simulink model "DSPB_MMSE"  (Simulink 8.1)
settings: Solver=VariableStepDiscrete  StartTime=0.0  StopTime=DSPB_MMSE_param.endTime  RelTol=1e-3
PreLoadFcn:
  | % Run the setup script when the model is opened
  | setup_DSPB_MMSE;
InitFcn:
  | % Run the setup script again just before the
  | % model is run, so that any updates made
  | % after opening are applied.
  | setup_DSPB_MMSE;
  | %% DSPBuilder Start
  | alt_dspbuilder_update_model(bdroot)
  | %% DSPBuilder End
StartFcn:
  | %% DSPBuilder Start
  | alt_dspbuilder_hdlimport_prepare_for_simulation(bdroot)
  | %% DSPBuilder End
undefined symbols (not defined in the file or in its folder): a, AdvDSPBDMemDisplay, dpoly, DSPB_MMSE_param, dspba, evalAionMaskParam, pow, primtype, UseDontCare, value, x, y
libraries: DSPBAPrim x213, DspbAdvFftLibrary x9, DSPBABase x5, simulink x3, DSPBAModelBus x3, DSPBAControl x1, DSPBAVectorUtil x1
(part 2 of 3)

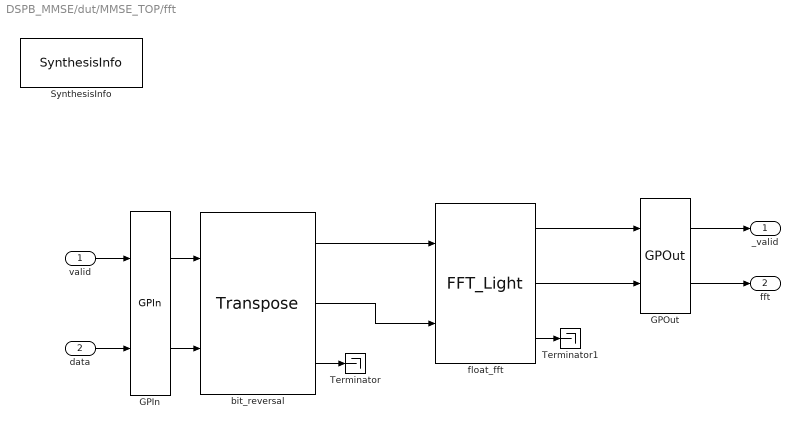
== system DSPB_MMSE/dut/MMSE_TOP/fft ==
  valid : Inport
  data : Inport  Port=2
  GPIn : DSPBAPrim/GPIn  primtype=gpin  nInputs=evalAionMaskParam(gcb,'value',1)  nOutputs=evalAionMaskParam(gcb,'value',1)  omode=Inherit via internal rule  otype=sfix(16)  scale=2^-15  rndmethod=Unbiased  factor=1  satmethod=Symmetric  shift_vec=[0 1 2 -1]  value=2  inPortNames=[' ' ' ' ' ' ' ' ' ' ' ' ' ' ' ' ' ' ' ' ' ' ' ' ' ' ' ' ' ' ' ' ' ' ' ' ' ' ' ' ' ' ' ' ' ' ' ' ' ' ' ' ' ' ' ' ' ' ' ' ' ' ' ' ' ' ' ' ' ']'  outPortNames=[' ' ' ' ' ' ' ' ' ' ' ' ' ' ' ' ' ' ' ' ' ' ' ' ' ' ' ' ' ' ' ' ' ' ' ' ' ' ' ' ' ' ' ' ' ' ' ' ' ' ' ' ' ' ' ' ' ' ' ' ' ' ' ' ' ' ' ' ' ']'  dspbaimage=dspba_prim.jpg  text=fprintf('GPIn');  style=Optimised  visibilities=1024  latencyCorrection=0  scheduleOrigin=on  version=20090407
  GPOut : DSPBAPrim/GPOut  primtype=gpout  nInputs=evalAionMaskParam(gcb,'value',1)  nOutputs=evalAionMaskParam(gcb,'value',1)  omode=Inherit via internal rule  otype=sfix(16)  scale=2^-15  rndmethod=Unbiased  factor=1  satmethod=Symmetric  shift_vec=[0 1 2 -1]  value=2  inPortNames=[' ' ' ' ' ' ' ' ' ' ' ' ' ' ' ' ' ' ' ' ' ' ' ' ' ' ' ' ' ' ' ' ' ' ' ' ' ' ' ' ' ' ' ' ' ' ' ' ' ' ' ' ' ' ' ' ' ' ' ' ' ' ' ' ' ' ' ' ' ']'  outPortNames=[' ' ' ' ' ' ' ' ' ' ' ' ' ' ' ' ' ' ' ' ' ' ' ' ' ' ' ' ' ' ' ' ' ' ' ' ' ' ' ' ' ' ' ' ' ' ' ' ' ' ' ' ' ' ' ' ' ' ' ' ' ' ' ' ' ' ' ' ' ']'  dspbaimage=dspba_prim.jpg  text=fprintf('GPOut');  style=Optimised  visibilities=1024  latencyCorrection=0  version=20090407
  SynthesisInfo : DSPBAPrim/SynthesisInfo  primtype=synthinfo  nInputs=0  nOutputs=0  omode=Inherit via internal rule  otype=sfix(16)  scale=2^-15  rndmethod=Truncate  factor=1  satmethod=Symmetric  shift_vec=[0 1 2 -1]  value=99  inPortNames=[' '; ' ';]  outPortNames=[' ']  dspbaimage=dspba_prim_ctrl.jpg  text=fprintf('Style=%s', style);  style=Scheduled  visibilities=32768  constraintInUse=off  constraintRelation=>  constraintLimit=2  bitAccurate=on  version=20150220
  Terminator : Terminator
  Terminator1 : Terminator
  bit_reversal : DspbAdvFftLibrary/Common/Transpose  perm=[fliplr(0:DSPB_MMSE_param.FS-1)]
  float_fft : DspbAdvFftLibrary/Common/FFT_Light  IFFT=false  subchannels=1  br_in=true  N=DSPB_MMSE_param.FS  in_type=dspba.namedVPFloat('single')  type_strings=dspba.fft.all_float(DSPB_MMSE_param.FS,dspba.namedVPFloat('single'))  faithful=false  wirecount=1
  _valid : Outport
  fft : Outport  Port=2
  wires:
  bit_reversal/3 -> Terminator/1
  bit_reversal/1 -> float_fft/1
  bit_reversal/2 -> float_fft/2
  float_fft/3 -> Terminator1/1
  GPIn/1 -> bit_reversal/1
  GPIn/2 -> bit_reversal/2
  valid/1 -> GPIn/1
  data/1 -> GPIn/2
  GPOut/1 -> _valid/1
  GPOut/2 -> fft/1
  float_fft/1 -> GPOut/1
  float_fft/2 -> GPOut/2

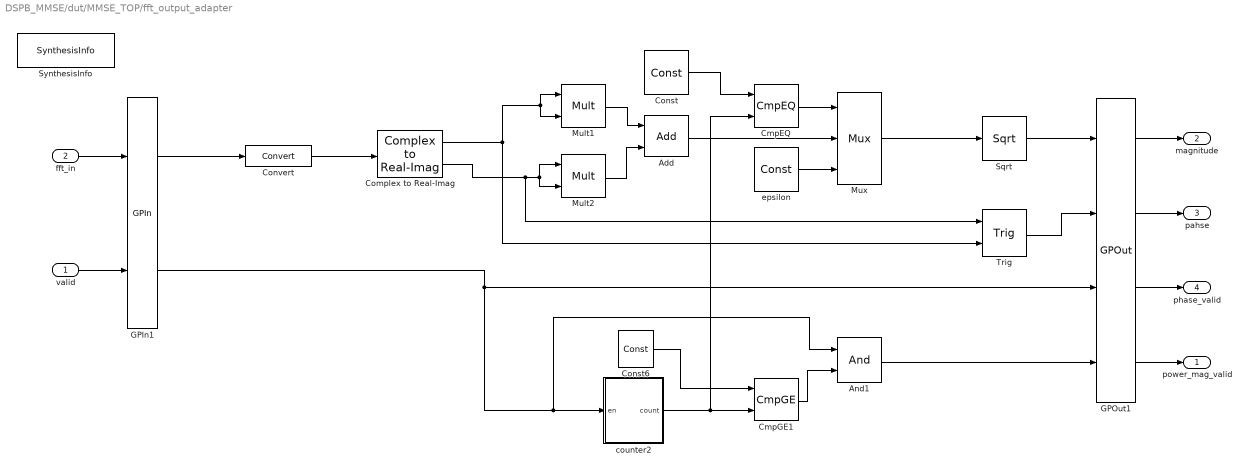
== system DSPB_MMSE/dut/MMSE_TOP/fft_output_adapter ==
  valid : Inport
  fft_in : Inport  Port=2
  Add : DSPBAPrim/Add  primtype=add  nInputs=evalAionMaskParam(gcb,'value',1)  nOutputs=1  omode=Inherit via internal rule with word growth  otype=sfix(16)  scale=2^-15  rndmethod=Unbiased  factor=1  satmethod=Symmetric  shift_vec=[0 1 2 -1]  value=2  inPortNames=[' '; ' ';]  outPortNames=[' ']  dspbaimage=dspba_prim.jpg  text=fprintf('+');  style=Optimised  visibilities=1032+2^17+2^18+2^19  genFPC=off  floatRounding=correct  advOptions=[]  version=20130821
  And1 : DSPBAPrim/And  primtype=and  nInputs=2  nOutputs=1  omode=Inherit via internal rule  otype=sfix(16)  scale=2^-15  rndmethod=Unbiased  factor=1  satmethod=Symmetric  shift_vec=[0 1 2 -1]  value=0  inPortNames=[' '; ' '; ' '; ' '; ' '; ' '; ' '; ' '; ' '; ' '; ' '; ' '; ' '; ' '; ' '; ' '; ]  outPortNames=[' ']  dspbaimage=dspba_prim.jpg  text=fprintf('&');  style=Optimised  visibilities=8+2  version=20090407
  CmpEQ : DSPBAPrim/CmpEQ  primtype=cmpeq  nInputs=2  nOutputs=1  omode=boolean  otype=sfix(16)  scale=2^-15  rndmethod=Unbiased  factor=1  satmethod=Symmetric  shift_vec=[0 1 2 -1]  value=0  inPortNames=[' '; ' ';]  outPortNames=[' ']  dspbaimage=dspba_prim.jpg  text=fprintf('==');  style=Optimised  visibilities=0  advOptions=[]  version=20130117
  CmpGE1 : DSPBAPrim/CmpGE  primtype=cmpgte  nInputs=2  nOutputs=1  omode=boolean  otype=sfix(16)  scale=2^-15  rndmethod=Unbiased  factor=1  satmethod=Symmetric  shift_vec=[0 1 2 -1]  value=0  inPortNames=['a'; 'b';]  outPortNames=[' ']  dspbaimage=dspba_prim.jpg  text=fprintf('a>=b');  style=Optimised  visibilities=0  advOptions=[]  version=20130117
  Complex to Real-Imag : DSPBAVectorUtil/Complex to Real-Imag
  Const : DSPBAPrim/Const  primtype=const  nInputs=0  nOutputs=1  omode=Inherit via internal rule  otype=sfix(16)  scale=2^-15  rndmethod=Unbiased  factor=1  satmethod=Symmetric  shift_vec=[0 1 2 -1]  value=1  inPortNames=['+'; '+';]  outPortNames=[' ']  dspbaimage=dspba_prim.jpg  text=fprintf('%s', num2str(value));  style=Optimised  visibilities=8 + 1024  floatPrecision=float32_m23  version=20120820
  Const6 : DSPBAPrim/Const  primtype=const  nInputs=0  nOutputs=1  omode=Specify via dialog  otype=ufix(DSPB_MMSE_param.FS+1)  scale=2^-0  rndmethod=Unbiased  factor=1  satmethod=Symmetric  shift_vec=[0 1 2 -1]  value=2^(DSPB_MMSE_param.FS-1)  inPortNames=['+'; '+';]  outPortNames=[' ']  dspbaimage=dspba_prim.jpg  text=fprintf('%s', num2str(value));  style=Optimised  visibilities=8 + 1024  floatPrecision=float32_m23  version=20120820
  Convert : DSPBAPrim/Convert  primtype=convert  nInputs=1  nOutputs=1  omode=single  otype=sfix(16)  scale=2^-15  rndmethod=Biased  factor=1  satmethod=None  shift_vec=[0 1 2 -1]  value=round([0:255]/17)  inPortNames=[' '; ' ';]  outPortNames=[' '; 'c']  dspbaimage=dspba_prim.jpg  text=fprintf('convert');  style=Optimised  visibilities=8+64+256+2^17  clipdetect=off  floatPrecision=float32_m23  advOptions=[]  version=20130211
  GPIn1 : DSPBAPrim/GPIn  primtype=gpin  nInputs=evalAionMaskParam(gcb,'value',1)  nOutputs=evalAionMaskParam(gcb,'value',1)  omode=Inherit via internal rule  otype=sfix(16)  scale=2^-15  rndmethod=Unbiased  factor=1  satmethod=Symmetric  shift_vec=[0 1 2 -1]  value=2  inPortNames=[' ' ' ' ' ' ' ' ' ' ' ' ' ' ' ' ' ' ' ' ' ' ' ' ' ' ' ' ' ' ' ' ' ' ' ' ' ' ' ' ' ' ' ' ' ' ' ' ' ' ' ' ' ' ' ' ' ' ' ' ' ' ' ' ' ' ' ' ' ']'  outPortNames=[' ' ' ' ' ' ' ' ' ' ' ' ' ' ' ' ' ' ' ' ' ' ' ' ' ' ' ' ' ' ' ' ' ' ' ' ' ' ' ' ' ' ' ' ' ' ' ' ' ' ' ' ' ' ' ' ' ' ' ' ' ' ' ' ' ' ' ' ' ']'  dspbaimage=dspba_prim.jpg  text=fprintf('GPIn');  style=Optimised  visibilities=1024  latencyCorrection=0  scheduleOrigin=on  version=20090407
  GPOut1 : DSPBAPrim/GPOut  primtype=gpout  nInputs=evalAionMaskParam(gcb,'value',1)  nOutputs=evalAionMaskParam(gcb,'value',1)  omode=Inherit via internal rule  otype=sfix(16)  scale=2^-15  rndmethod=Unbiased  factor=1  satmethod=Symmetric  shift_vec=[0 1 2 -1]  value=4  inPortNames=[' ' ' ' ' ' ' ' ' ' ' ' ' ' ' ' ' ' ' ' ' ' ' ' ' ' ' ' ' ' ' ' ' ' ' ' ' ' ' ' ' ' ' ' ' ' ' ' ' ' ' ' ' ' ' ' ' ' ' ' ' ' ' ' ' ' ' ' ' ']'  outPortNames=[' ' ' ' ' ' ' ' ' ' ' ' ' ' ' ' ' ' ' ' ' ' ' ' ' ' ' ' ' ' ' ' ' ' ' ' ' ' ' ' ' ' ' ' ' ' ' ' ' ' ' ' ' ' ' ' ' ' ' ' ' ' ' ' ' ' ' ' ' ']'  dspbaimage=dspba_prim.jpg  text=fprintf('GPOut');  style=Optimised  visibilities=1024  latencyCorrection=0  version=20090407
  Mult1 : DSPBAPrim/Mult  primtype=mult  nInputs=2  nOutputs=1  omode=Inherit via internal rule  otype=sfix(16)  scale=2^-15  rndmethod=Unbiased  factor=1  satmethod=Symmetric  shift_vec=[0 1 2 -1]  value=0  inPortNames=[' '; ' ';]  outPortNames=[' ']  dspbaimage=dspba_prim.jpg  text=fprintf('X');  style=Optimised  visibilities=8+2^18+2^19  floatPrecision=float32_m23  floatRounding=correct  advOptions=[]  version=20130115
  Mult2 : DSPBAPrim/Mult  primtype=mult  nInputs=2  nOutputs=1  omode=Inherit via internal rule  otype=sfix(16)  scale=2^-15  rndmethod=Unbiased  factor=1  satmethod=Symmetric  shift_vec=[0 1 2 -1]  value=0  inPortNames=[' '; ' ';]  outPortNames=[' ']  dspbaimage=dspba_prim.jpg  text=fprintf('X');  style=Optimised  visibilities=8+2^18+2^19  floatPrecision=float32_m23  floatRounding=correct  advOptions=[]  version=20130115
  Mux : DSPBAPrim/Mux  primtype=mux  nInputs=evalAionMaskParam(gcb,'value',1)+1  nOutputs=1  omode=Inherit via internal rule  otype=sfix(16)  scale=2^-15  rndmethod=Unbiased  factor=1  satmethod=Symmetric  shift_vec=[0 1 2 -1]  value=2  inPortNames=['s '; 'd0'; 'd1'; 'd2'; 'd3'; 'd4'; 'd5'; 'd6'; 'd7'; 'd8'; 'd9';]  outPortNames=[' ']  dspbaimage=dspba_prim.jpg  text=fprintf('%s', primtype);  style=Optimised  visibilities=1032  version=20131025
  Sqrt : DSPBAPrim/Sqrt  primtype=sqrtfunc  nInputs=1  nOutputs=1  omode=Inherit via internal rule  otype=sfix(16)  scale=2^-15  rndmethod=Unbiased  factor=1  satmethod=Symmetric  shift_vec=[0 1 2 -1]  value=round([0:255]/17)  inPortNames=[' '; ' ';]  outPortNames=[' ']  dspbaimage=dspba_prim_float.jpg  text=fprintf('sqrt(x)');  style=Optimised  visibilities=2^17  functionExpr=sqrt(x)  floatRounding=correct  advOptions=[]  version=20120730
  SynthesisInfo : DSPBAPrim/SynthesisInfo  primtype=synthinfo  nInputs=0  nOutputs=0  omode=Inherit via internal rule  otype=sfix(16)  scale=2^-15  rndmethod=Truncate  factor=1  satmethod=Symmetric  shift_vec=[0 1 2 -1]  value=99  inPortNames=[' '; ' ';]  outPortNames=[' ']  dspbaimage=dspba_prim_ctrl.jpg  text=fprintf('Style=%s', style);  style=Scheduled  visibilities=2^17+2^18+2^19+2^20  constraintInUse=off  constraintRelation=>  constraintLimit=2  bitAccurate=on  version=20150220
  Trig : DSPBAPrim/Trig  primtype=trigfunc  nInputs=1  nOutputs=1  omode=Inherit via internal rule  otype=sfix(16)  scale=2^-15  rndmethod=Unbiased  factor=1  satmethod=Symmetric  shift_vec=[0 1 2 -1]  value=round([0:255]/17)  inPortNames=[' '; ' ';]  outPortNames=[' ']  dspbaimage=dspba_prim_float.jpg  text=fprintf('sin(a)');  style=Optimised  visibilities=2^17+2^18  functionExpr=atan2(y;x)  advOptions=[]  version=20140803
  counter2 : Subsystem
  epsilon : DSPBAPrim/Const  primtype=const  nInputs=0  nOutputs=1  omode=single  otype=sfix(16)  scale=2^-15  rndmethod=Unbiased  factor=1  satmethod=Symmetric  shift_vec=[0 1 2 -1]  value=2^-126  inPortNames=['+'; '+';]  outPortNames=[' ']  dspbaimage=dspba_prim.jpg  text=fprintf('%s', num2str(value));  style=Optimised  visibilities=8 + 1024  floatPrecision=float32_m23  version=20120820
  power_mag_valid : Outport
  magnitude : Outport  Port=2
  pahse : Outport  Port=3
  phase_valid : Outport  Port=4
  wires:
  Mult1/1 -> Add/1
  Mult2/1 -> Add/2
  GPOut1/1 -> magnitude/1
  valid/1 -> GPIn1/2
  fft_in/1 -> GPIn1/1
  GPIn1/1 -> Convert/1
  GPOut1/2 -> pahse/1
  Complex to Real-Imag/1 -> Mult1/2, Mult1/1, Trig/2
  Complex to Real-Imag/2 -> Trig/1, Mult2/2, Mult2/1
  GPOut1/3 -> phase_valid/1
  Trig/1 -> GPOut1/2
  GPIn1/2 -> counter2/1(en), And1/1, GPOut1/3
  Const6/1 -> CmpGE1/1
  counter2/1(count) -> CmpEQ/2, CmpGE1/2
  CmpGE1/1 -> And1/2
  And1/1 -> GPOut1/4
  GPOut1/4 -> power_mag_valid/1
  Mux/1 -> Sqrt/1
  Sqrt/1 -> GPOut1/1
  Convert/1 -> Complex to Real-Imag/1
  Const/1 -> CmpEQ/1
  CmpEQ/1 -> Mux/1
  Add/1 -> Mux/2
  epsilon/1 -> Mux/3

== system DSPB_MMSE/dut/MMSE_TOP/reconstruct ==
  valid : Inport
  enhanced_mag : Inport  Port=2
  phase : Inport  Port=3
  pahse_valid : Inport  Port=4
  ifft : Subsystem
  ifft_input_adapter : Subsystem
  _valid : Outport
  output : Outport  Port=2
  wires:
  ifft/2(ifft) -> output/1
  valid/1 -> ifft_input_adapter/2(valid)
  ifft/1(_valid) -> _valid/1
  ifft_input_adapter/1(_valid) -> ifft/1(valid)
  ifft_input_adapter/2(out) -> ifft/2(data)
  enhanced_mag/1 -> ifft_input_adapter/3(enhanced_mag)
  pahse_valid/1 -> ifft_input_adapter/1(phase_valid)
  phase/1 -> ifft_input_adapter/4(phase)

== system DSPB_MMSE/dut/MM_in/addr_counter ==
  en : Inport
  CmpEQ : DSPBAPrim/CmpEQ  primtype=cmpeq  nInputs=2  nOutputs=1  omode=boolean  otype=sfix(16)  scale=2^-15  rndmethod=Unbiased  factor=1  satmethod=Symmetric  shift_vec=[0 1 2 -1]  value=0  inPortNames=[' '; ' ';]  outPortNames=[' ']  dspbaimage=dspba_prim.jpg  text=fprintf('==');  style=Optimised  visibilities=0  advOptions=[]  version=20130117
  Const1 : DSPBAPrim/Const  primtype=const  nInputs=0  nOutputs=1  omode=Specify via dialog  otype=ufix(DSPB_MMSE_param.FS+1)  scale=2^-0  rndmethod=Unbiased  factor=1  satmethod=Symmetric  shift_vec=[0 1 2 -1]  value=2^(DSPB_MMSE_param.FS) + 1  inPortNames=['+'; '+';]  outPortNames=[' ']  dspbaimage=dspba_prim.jpg  text=fprintf('%s', num2str(value));  style=Optimised  visibilities=8 + 1024  floatPrecision=float32_m23  version=20120820
  Const2 : DSPBAPrim/Const  primtype=const  nInputs=0  nOutputs=1  omode=Specify via dialog  otype=ufix(DSPB_MMSE_param.FS + 1)  scale=2^-0  rndmethod=Unbiased  factor=1  satmethod=Symmetric  shift_vec=[0 1 2 -1]  value=2^(DSPB_MMSE_param.FS)  inPortNames=['+'; '+';]  outPortNames=[' ']  dspbaimage=dspba_prim.jpg  text=fprintf('%s', num2str(value));  style=Optimised  visibilities=8 + 1024  floatPrecision=float32_m23  version=20120820
  Const3 : DSPBAPrim/Const  primtype=const  nInputs=0  nOutputs=1  omode=boolean  otype=ufix(10)  scale=2^-0  rndmethod=Unbiased  factor=1  satmethod=Symmetric  shift_vec=[0 1 2 -1]  value=1  inPortNames=['+'; '+';]  outPortNames=[' ']  dspbaimage=dspba_prim.jpg  text=fprintf('%s', num2str(value));  style=Optimised  visibilities=8 + 1024  floatPrecision=float32_m23  version=20120820
  Const4 : DSPBAPrim/Const  primtype=const  nInputs=0  nOutputs=1  omode=Inherit via internal rule  otype=ufix(10)  scale=2^-0  rndmethod=Unbiased  factor=1  satmethod=Symmetric  shift_vec=[0 1 2 -1]  value=0  inPortNames=['+'; '+';]  outPortNames=[' ']  dspbaimage=dspba_prim.jpg  text=fprintf('%s', num2str(value));  style=Optimised  visibilities=8 + 1024  floatPrecision=float32_m23  version=20120820
  LoadableCounter : DSPBAPrim/LoadableCounter  primtype=loadablecounter  nInputs=5  nOutputs=1  omode=Specify via dialog  otype=ufix(DSPB_MMSE_param.FS+1)  scale=2^-0  rndmethod=Unbiased  factor=1  satmethod=Symmetric  shift_vec=[0 1 2 -1]  value=[0 2^(DSPB_MMSE_param.FS) + 1 1]  inPortNames=['en';'ld';'i ';'s ';'m ']  outPortNames=[' ']  dspbaimage=dspba_prim.jpg  text=fprintf('loadable\ncounter\n[%d %d %d]', value(1), value(2), value(3));  style=Optimised  visibilities=8 + 1024  version=20090407
  SampleDelay : DSPBAPrim/SampleDelay  primtype=sampdelay  nInputs=1  nOutputs=1  omode=Inherit via internal rule  otype=sfix(16)  scale=2^-15  rndmethod=Unbiased  factor=1  satmethod=Symmetric  shift_vec=[0 1 2 -1]  value=1  inPortNames=[' '; ' ';]  outPortNames=[' ']  dspbaimage=dspba_prim.jpg  text=dpoly(1, eye(1,value+1), 'z')  style=Optimised  visibilities=8 + 1024 + 2^17 + 2^18  flexible=off  slackgroup=0  augmented=0  version=20090407  advOptions=[]
  count : Outport
  wires:
  Const2/1 -> CmpEQ/2
  CmpEQ/1 -> SampleDelay/1
  Const4/1 -> LoadableCounter/3
  Const1/1 -> LoadableCounter/5
  SampleDelay/1 -> LoadableCounter/2
  Const3/1 -> LoadableCounter/4
  en/1 -> LoadableCounter/1
  LoadableCounter/1 -> count/1, CmpEQ/1

== system DSPB_MMSE/dut/MM_out/addr_counter1 ==
  en : Inport
  CmpEQ : DSPBAPrim/CmpEQ  primtype=cmpeq  nInputs=2  nOutputs=1  omode=boolean  otype=sfix(16)  scale=2^-15  rndmethod=Unbiased  factor=1  satmethod=Symmetric  shift_vec=[0 1 2 -1]  value=0  inPortNames=[' '; ' ';]  outPortNames=[' ']  dspbaimage=dspba_prim.jpg  text=fprintf('==');  style=Optimised  visibilities=0  advOptions=[]  version=20130117
  Const1 : DSPBAPrim/Const  primtype=const  nInputs=0  nOutputs=1  omode=Specify via dialog  otype=ufix(DSPB_MMSE_param.FS+1)  scale=2^-0  rndmethod=Unbiased  factor=1  satmethod=Symmetric  shift_vec=[0 1 2 -1]  value=2^(DSPB_MMSE_param.FS) + 1  inPortNames=['+'; '+';]  outPortNames=[' ']  dspbaimage=dspba_prim.jpg  text=fprintf('%s', num2str(value));  style=Optimised  visibilities=8 + 1024  floatPrecision=float32_m23  version=20120820
  Const2 : DSPBAPrim/Const  primtype=const  nInputs=0  nOutputs=1  omode=Specify via dialog  otype=ufix(DSPB_MMSE_param.FS + 1)  scale=2^-0  rndmethod=Unbiased  factor=1  satmethod=Symmetric  shift_vec=[0 1 2 -1]  value=2^(DSPB_MMSE_param.FS)  inPortNames=['+'; '+';]  outPortNames=[' ']  dspbaimage=dspba_prim.jpg  text=fprintf('%s', num2str(value));  style=Optimised  visibilities=8 + 1024  floatPrecision=float32_m23  version=20120820
  Const3 : DSPBAPrim/Const  primtype=const  nInputs=0  nOutputs=1  omode=boolean  otype=ufix(10)  scale=2^-0  rndmethod=Unbiased  factor=1  satmethod=Symmetric  shift_vec=[0 1 2 -1]  value=1  inPortNames=['+'; '+';]  outPortNames=[' ']  dspbaimage=dspba_prim.jpg  text=fprintf('%s', num2str(value));  style=Optimised  visibilities=8 + 1024  floatPrecision=float32_m23  version=20120820
  Const4 : DSPBAPrim/Const  primtype=const  nInputs=0  nOutputs=1  omode=Inherit via internal rule  otype=ufix(10)  scale=2^-0  rndmethod=Unbiased  factor=1  satmethod=Symmetric  shift_vec=[0 1 2 -1]  value=0  inPortNames=['+'; '+';]  outPortNames=[' ']  dspbaimage=dspba_prim.jpg  text=fprintf('%s', num2str(value));  style=Optimised  visibilities=8 + 1024  floatPrecision=float32_m23  version=20120820
  LoadableCounter : DSPBAPrim/LoadableCounter  primtype=loadablecounter  nInputs=5  nOutputs=1  omode=Specify via dialog  otype=ufix(DSPB_MMSE_param.FS+1)  scale=2^-0  rndmethod=Unbiased  factor=1  satmethod=Symmetric  shift_vec=[0 1 2 -1]  value=[0 2^(DSPB_MMSE_param.FS) + 1 1]  inPortNames=['en';'ld';'i ';'s ';'m ']  outPortNames=[' ']  dspbaimage=dspba_prim.jpg  text=fprintf('loadable\ncounter\n[%d %d %d]', value(1), value(2), value(3));  style=Optimised  visibilities=8 + 1024  version=20090407
  SampleDelay : DSPBAPrim/SampleDelay  primtype=sampdelay  nInputs=1  nOutputs=1  omode=Inherit via internal rule  otype=sfix(16)  scale=2^-15  rndmethod=Unbiased  factor=1  satmethod=Symmetric  shift_vec=[0 1 2 -1]  value=1  inPortNames=[' '; ' ';]  outPortNames=[' ']  dspbaimage=dspba_prim.jpg  text=dpoly(1, eye(1,value+1), 'z')  style=Optimised  visibilities=8 + 1024 + 2^17 + 2^18  flexible=off  slackgroup=0  augmented=0  version=20090407  advOptions=[]
  count : Outport
  wires:
  Const2/1 -> CmpEQ/2
  CmpEQ/1 -> SampleDelay/1
  Const4/1 -> LoadableCounter/3
  Const1/1 -> LoadableCounter/5
  SampleDelay/1 -> LoadableCounter/2
  Const3/1 -> LoadableCounter/4
  en/1 -> LoadableCounter/1
  LoadableCounter/1 -> count/1, CmpEQ/1

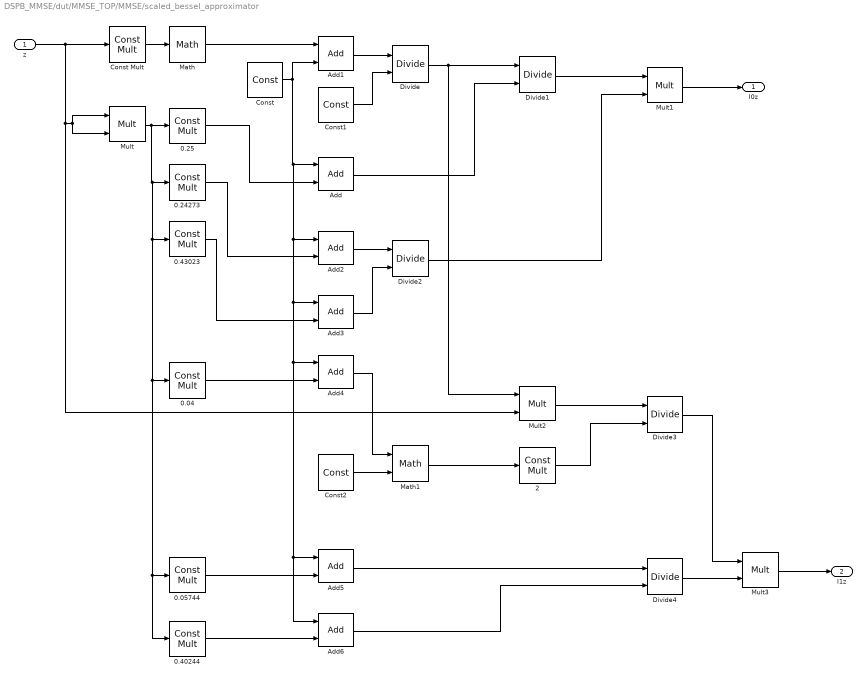
== system DSPB_MMSE/dut/MMSE_TOP/MMSE/scaled_bessel_approximator ==
  z : Inport
  0.04 : DSPBAPrim/Const Mult  primtype=constmult  nInputs=1  nOutputs=1  omode=Inherit via internal rule  otype=sfix(16)  scale=2^-15  rndmethod=Unbiased  factor=1  satmethod=Symmetric  shift_vec=[0 1 2 -1]  value=0.04  inPortNames=[' '; ' ';]  outPortNames=[' ']  dspbaimage=dspba_prim.jpg  text=fprintf('cx');  style=Optimised  visibilities=8+2^10+2^17+2^18  floatRounding=faithful  advOptions=[]  version=20140218
  0.05744 : DSPBAPrim/Const Mult  primtype=constmult  nInputs=1  nOutputs=1  omode=Inherit via internal rule  otype=sfix(16)  scale=2^-15  rndmethod=Unbiased  factor=1  satmethod=Symmetric  shift_vec=[0 1 2 -1]  value=0.05744  inPortNames=[' '; ' ';]  outPortNames=[' ']  dspbaimage=dspba_prim.jpg  text=fprintf('cx');  style=Optimised  visibilities=8+2^10+2^17+2^18  floatRounding=faithful  advOptions=[]  version=20140218
  0.24273 : DSPBAPrim/Const Mult  primtype=constmult  nInputs=1  nOutputs=1  omode=Inherit via internal rule  otype=sfix(16)  scale=2^-15  rndmethod=Unbiased  factor=1  satmethod=Symmetric  shift_vec=[0 1 2 -1]  value=0.24273  inPortNames=[' '; ' ';]  outPortNames=[' ']  dspbaimage=dspba_prim.jpg  text=fprintf('cx');  style=Optimised  visibilities=8+2^10+2^17+2^18  floatRounding=faithful  advOptions=[]  version=20140218
  0.25 : DSPBAPrim/Const Mult  primtype=constmult  nInputs=1  nOutputs=1  omode=Inherit via internal rule  otype=sfix(16)  scale=2^-15  rndmethod=Unbiased  factor=1  satmethod=Symmetric  shift_vec=[0 1 2 -1]  value=0.25  inPortNames=[' '; ' ';]  outPortNames=[' ']  dspbaimage=dspba_prim.jpg  text=fprintf('cx');  style=Optimised  visibilities=8+2^10+2^17+2^18  floatRounding=faithful  advOptions=[]  version=20140218
  0.40244 : DSPBAPrim/Const Mult  primtype=constmult  nInputs=1  nOutputs=1  omode=Inherit via internal rule  otype=sfix(16)  scale=2^-15  rndmethod=Unbiased  factor=1  satmethod=Symmetric  shift_vec=[0 1 2 -1]  value=0.40244  inPortNames=[' '; ' ';]  outPortNames=[' ']  dspbaimage=dspba_prim.jpg  text=fprintf('cx');  style=Optimised  visibilities=8+2^10+2^17+2^18  floatRounding=faithful  advOptions=[]  version=20140218
  0.43023 : DSPBAPrim/Const Mult  primtype=constmult  nInputs=1  nOutputs=1  omode=Inherit via internal rule  otype=sfix(16)  scale=2^-15  rndmethod=Unbiased  factor=1  satmethod=Symmetric  shift_vec=[0 1 2 -1]  value=0.43023  inPortNames=[' '; ' ';]  outPortNames=[' ']  dspbaimage=dspba_prim.jpg  text=fprintf('cx');  style=Optimised  visibilities=8+2^10+2^17+2^18  floatRounding=faithful  advOptions=[]  version=20140218
  2 : DSPBAPrim/Const Mult  primtype=constmult  nInputs=1  nOutputs=1  omode=Inherit via internal rule  otype=sfix(16)  scale=2^-15  rndmethod=Unbiased  factor=1  satmethod=Symmetric  shift_vec=[0 1 2 -1]  value=2  inPortNames=[' '; ' ';]  outPortNames=[' ']  dspbaimage=dspba_prim.jpg  text=fprintf('cx');  style=Optimised  visibilities=8+2^10+2^17+2^18  floatRounding=faithful  advOptions=[]  version=20140218
  Add{,1..6} (7 alike) : DSPBAPrim/Add  primtype=add  nInputs=evalAionMaskParam(gcb,'value',1)  nOutputs=1  omode=Inherit via internal rule with word growth  otype=sfix(16)  scale=2^-15  rndmethod=Unbiased  factor=1  satmethod=Symmetric  shift_vec=[0 1 2 -1]  value=2  inPortNames=[' '; ' ';]  outPortNames=[' ']  dspbaimage=dspba_prim.jpg  text=fprintf('+');  style=Optimised  visibilities=1032+2^17+2^18+2^19  genFPC=on  floatRounding=faithful  advOptions=[]  version=20130821
  Const : DSPBAPrim/Const  primtype=const  nInputs=0  nOutputs=1  omode=single  otype=sfix(16)  scale=2^-15  rndmethod=Unbiased  factor=1  satmethod=Symmetric  shift_vec=[0 1 2 -1]  value=1  inPortNames=['+'; '+';]  outPortNames=[' ']  dspbaimage=dspba_prim.jpg  text=fprintf('%s', num2str(value));  style=Optimised  visibilities=8 + 1024  floatPrecision=float32_m23  version=20120820
  Const Mult : DSPBAPrim/Const Mult  primtype=constmult  nInputs=1  nOutputs=1  omode=Inherit via internal rule  otype=sfix(16)  scale=2^-15  rndmethod=Unbiased  factor=1  satmethod=Symmetric  shift_vec=[0 1 2 -1]  value=-2  inPortNames=[' '; ' ';]  outPortNames=[' ']  dspbaimage=dspba_prim.jpg  text=fprintf('cx');  style=Optimised  visibilities=8+2^10+2^17+2^18  floatRounding=faithful  advOptions=[]  version=20140218
  Const1 : DSPBAPrim/Const  primtype=const  nInputs=0  nOutputs=1  omode=single  otype=sfix(16)  scale=2^-15  rndmethod=Unbiased  factor=1  satmethod=Symmetric  shift_vec=[0 1 2 -1]  value=2  inPortNames=['+'; '+';]  outPortNames=[' ']  dspbaimage=dspba_prim.jpg  text=fprintf('%s', num2str(value));  style=Optimised  visibilities=8 + 1024  floatPrecision=float32_m23  version=20120820
  Const2 : DSPBAPrim/Const  primtype=const  nInputs=0  nOutputs=1  omode=single  otype=sfix(16)  scale=2^-15  rndmethod=Unbiased  factor=1  satmethod=Symmetric  shift_vec=[0 1 2 -1]  value=3/4  inPortNames=['+'; '+';]  outPortNames=[' ']  dspbaimage=dspba_prim.jpg  text=fprintf('%s', num2str(value));  style=Optimised  visibilities=8 + 1024  floatPrecision=float32_m23  version=20120820
  Divide{,1..4} (5 alike) : DSPBAPrim/Divide  primtype=divide  nInputs=2  nOutputs=1  omode=Inherit via internal rule  otype=sfix(16)  scale=2^-15  rndmethod=Unbiased  factor=1  satmethod=Symmetric  shift_vec=[0 1 2 -1]  value=round([0:255]/17)  inPortNames=[' '; ' ';]  outPortNames=[' ']  dspbaimage=dspba_prim.jpg  text=fprintf('a\n----\nb');  style=Optimised  visibilities=8+2^17+2^18  floatRounding=faithful  advOptions=[]  version=20130115
  Math : DSPBAPrim/Math  primtype=mathfunc  nInputs=1  nOutputs=1  omode=Inherit via internal rule  otype=sfix(16)  scale=2^-15  rndmethod=Unbiased  factor=1  satmethod=Symmetric  shift_vec=[0 1 2 -1]  value=round([0:255]/17)  inPortNames=[' '; ' ';]  outPortNames=[' ']  dspbaimage=dspba_prim_float.jpg  text=fprintf('exp(x)');  style=Optimised  visibilities=2^17  functionExpr=exp(x)  advOptions=[]  floatRounding=correct  version=20130910
  Math1 : DSPBAPrim/Math  primtype=mathfunc  nInputs=1  nOutputs=1  omode=Inherit via internal rule  otype=sfix(16)  scale=2^-15  rndmethod=Unbiased  factor=1  satmethod=Symmetric  shift_vec=[0 1 2 -1]  value=round([0:255]/17)  inPortNames=[' '; ' ';]  outPortNames=[' ']  dspbaimage=dspba_prim_float.jpg  text=fprintf('exp(x)');  style=Optimised  visibilities=2^17  functionExpr=pow(x;y)  advOptions=[]  floatRounding=correct  version=20130910
  Mult{,1..3} (4 alike) : DSPBAPrim/Mult  primtype=mult  nInputs=2  nOutputs=1  omode=Inherit via internal rule  otype=sfix(16)  scale=2^-15  rndmethod=Unbiased  factor=1  satmethod=Symmetric  shift_vec=[0 1 2 -1]  value=0  inPortNames=[' '; ' ';]  outPortNames=[' ']  dspbaimage=dspba_prim.jpg  text=fprintf('X');  style=Optimised  visibilities=8+2^18+2^19  floatPrecision=float32_m23  floatRounding=faithful  advOptions=[]  version=20130115
  I0z : Outport
  I1z : Outport  Port=2
  wires:
  z/1 -> Mult2/2, Mult/2, Mult/1, Const Mult/1
  Const Mult/1 -> Math/1
  Const/1 -> Add1/2, Add6/1, Add5/1, Add4/1, Add3/1, Add2/1, Add/1
  Math/1 -> Add1/1
  Add1/1 -> Divide/1
  Const1/1 -> Divide/2
  Divide/1 -> Mult2/1, Divide1/1
  Mult/1 -> 0.40244/1, 0.05744/1, 0.04/1, 0.43023/1, 0.24273/1, 0.25/1
  0.25/1 -> Add/2
  Add/1 -> Divide1/2
  Divide1/1 -> Mult1/1
  0.24273/1 -> Add2/2
  Add2/1 -> Divide2/1
  0.43023/1 -> Add3/2
  Add3/1 -> Divide2/2
  Divide2/1 -> Mult1/2
  Mult1/1 -> I0z/1
  Mult2/1 -> Divide3/1
  0.04/1 -> Add4/2
  Add4/1 -> Math1/1
  Const2/1 -> Math1/2
  Math1/1 -> 2/1
  2/1 -> Divide3/2
  Divide3/1 -> Mult3/1
  Divide4/1 -> Mult3/2
  0.05744/1 -> Add5/2
  0.40244/1 -> Add6/2
  Add5/1 -> Divide4/1
  Add6/1 -> Divide4/2
  Mult3/1 -> I1z/1

== system DSPB_MMSE/dut/MMSE_TOP/MMSE/v_k ==
  a_priori_snr : Inport
  a_posteriori_snr : Inport  Port=2
  Add : DSPBAPrim/Add  primtype=add  nInputs=evalAionMaskParam(gcb,'value',1)  nOutputs=1  omode=Inherit via internal rule with word growth  otype=sfix(16)  scale=2^-15  rndmethod=Unbiased  factor=1  satmethod=Symmetric  shift_vec=[0 1 2 -1]  value=2  inPortNames=[' '; ' ';]  outPortNames=[' ']  dspbaimage=dspba_prim.jpg  text=fprintf('+');  style=Optimised  visibilities=1032+2^17+2^18+2^19  genFPC=off  floatRounding=correct  advOptions=[]  version=20130821
  Const1 : DSPBAPrim/Const  primtype=const  nInputs=0  nOutputs=1  omode=single  otype=sfix(16)  scale=2^-15  rndmethod=Unbiased  factor=1  satmethod=Symmetric  shift_vec=[0 1 2 -1]  value=1  inPortNames=['+'; '+';]  outPortNames=[' ']  dspbaimage=dspba_prim.jpg  text=fprintf('%s', num2str(value));  style=Optimised  visibilities=8 + 1024  floatPrecision=float32_m23  version=20120820
  Divide1 : DSPBAPrim/Divide  primtype=divide  nInputs=2  nOutputs=1  omode=Inherit via internal rule  otype=sfix(16)  scale=2^-15  rndmethod=Unbiased  factor=1  satmethod=Symmetric  shift_vec=[0 1 2 -1]  value=round([0:255]/17)  inPortNames=[' '; ' ';]  outPortNames=[' ']  dspbaimage=dspba_prim.jpg  text=fprintf('a\n----\nb');  style=Optimised  visibilities=8+2^17+2^18  floatRounding=correct  advOptions=[]  version=20130115
  Mult1 : DSPBAPrim/Mult  primtype=mult  nInputs=2  nOutputs=1  omode=Inherit via internal rule  otype=sfix(16)  scale=2^-15  rndmethod=Unbiased  factor=1  satmethod=Symmetric  shift_vec=[0 1 2 -1]  value=0  inPortNames=[' '; ' ';]  outPortNames=[' ']  dspbaimage=dspba_prim.jpg  text=fprintf('X');  style=Optimised  visibilities=8+2^18+2^19  floatPrecision=float32_m23  floatRounding=correct  advOptions=[]  version=20130115
  v_k : Outport
  wires:
  a_priori_snr/1 -> Divide1/1, Add/1
  Const1/1 -> Add/2
  a_posteriori_snr/1 -> Mult1/2
  Add/1 -> Divide1/2
  Divide1/1 -> Mult1/1
  Mult1/1 -> v_k/1

== system DSPB_MMSE/dut/MMSE_TOP/a_posteriori_snr/counter ==
  en : Inport
  CmpEQ : DSPBAPrim/CmpEQ  primtype=cmpeq  nInputs=2  nOutputs=1  omode=boolean  otype=sfix(16)  scale=2^-15  rndmethod=Unbiased  factor=1  satmethod=Symmetric  shift_vec=[0 1 2 -1]  value=0  inPortNames=[' '; ' ';]  outPortNames=[' ']  dspbaimage=dspba_prim.jpg  text=fprintf('==');  style=Optimised  visibilities=0  advOptions=[]  version=20130117
  Const1 : DSPBAPrim/Const  primtype=const  nInputs=0  nOutputs=1  omode=Specify via dialog  otype=ufix(DSPB_MMSE_param.FS+1)  scale=2^-0  rndmethod=Unbiased  factor=1  satmethod=Symmetric  shift_vec=[0 1 2 -1]  value=2^(DSPB_MMSE_param.FS-1)+1  inPortNames=['+'; '+';]  outPortNames=[' ']  dspbaimage=dspba_prim.jpg  text=fprintf('%s', num2str(value));  style=Optimised  visibilities=8 + 1024  floatPrecision=float32_m23  version=20120820
  Const2 : DSPBAPrim/Const  primtype=const  nInputs=0  nOutputs=1  omode=Specify via dialog  otype=ufix(DSPB_MMSE_param.FS + 1)  scale=2^-0  rndmethod=Unbiased  factor=1  satmethod=Symmetric  shift_vec=[0 1 2 -1]  value=2^(DSPB_MMSE_param.FS-1)  inPortNames=['+'; '+';]  outPortNames=[' ']  dspbaimage=dspba_prim.jpg  text=fprintf('%s', num2str(value));  style=Optimised  visibilities=8 + 1024  floatPrecision=float32_m23  version=20120820
  Const3 : DSPBAPrim/Const  primtype=const  nInputs=0  nOutputs=1  omode=boolean  otype=ufix(10)  scale=2^-0  rndmethod=Unbiased  factor=1  satmethod=Symmetric  shift_vec=[0 1 2 -1]  value=1  inPortNames=['+'; '+';]  outPortNames=[' ']  dspbaimage=dspba_prim.jpg  text=fprintf('%s', num2str(value));  style=Optimised  visibilities=8 + 1024  floatPrecision=float32_m23  version=20120820
  Const4 : DSPBAPrim/Const  primtype=const  nInputs=0  nOutputs=1  omode=Inherit via internal rule  otype=ufix(10)  scale=2^-0  rndmethod=Unbiased  factor=1  satmethod=Symmetric  shift_vec=[0 1 2 -1]  value=0  inPortNames=['+'; '+';]  outPortNames=[' ']  dspbaimage=dspba_prim.jpg  text=fprintf('%s', num2str(value));  style=Optimised  visibilities=8 + 1024  floatPrecision=float32_m23  version=20120820
  LoadableCounter : DSPBAPrim/LoadableCounter  primtype=loadablecounter  nInputs=5  nOutputs=1  omode=Specify via dialog  otype=ufix(DSPB_MMSE_param.FS+1)  scale=2^-0  rndmethod=Unbiased  factor=1  satmethod=Symmetric  shift_vec=[0 1 2 -1]  value=[0 2^(DSPB_MMSE_param.FS-1)+1 1]  inPortNames=['en';'ld';'i ';'s ';'m ']  outPortNames=[' ']  dspbaimage=dspba_prim.jpg  text=fprintf('loadable\ncounter\n[%d %d %d]', value(1), value(2), value(3));  style=Optimised  visibilities=8 + 1024  version=20090407
  SampleDelay : DSPBAPrim/SampleDelay  primtype=sampdelay  nInputs=1  nOutputs=1  omode=Inherit via internal rule  otype=sfix(16)  scale=2^-15  rndmethod=Unbiased  factor=1  satmethod=Symmetric  shift_vec=[0 1 2 -1]  value=1  inPortNames=[' '; ' ';]  outPortNames=[' ']  dspbaimage=dspba_prim.jpg  text=dpoly(1, eye(1,value+1), 'z')  style=Optimised  visibilities=8 + 1024 + 2^17 + 2^18  flexible=off  slackgroup=0  augmented=0  version=20090407  advOptions=[]
  count : Outport
  wires:
  Const2/1 -> CmpEQ/2
  CmpEQ/1 -> SampleDelay/1
  Const4/1 -> LoadableCounter/3
  Const1/1 -> LoadableCounter/5
  SampleDelay/1 -> LoadableCounter/2
  Const3/1 -> LoadableCounter/4
  en/1 -> LoadableCounter/1
  LoadableCounter/1 -> CmpEQ/1, count/1

== system DSPB_MMSE/dut/MMSE_TOP/a_posteriori_snr/frame_fuse ==
  input : Inport
  CmpEQ : DSPBAPrim/CmpEQ  primtype=cmpeq  nInputs=2  nOutputs=1  omode=boolean  otype=sfix(16)  scale=2^-15  rndmethod=Unbiased  factor=1  satmethod=Symmetric  shift_vec=[0 1 2 -1]  value=0  inPortNames=[' '; ' ';]  outPortNames=[' ']  dspbaimage=dspba_prim.jpg  text=fprintf('==');  style=Optimised  visibilities=0  advOptions=[]  version=20130117
  Const : DSPBAPrim/Const  primtype=const  nInputs=0  nOutputs=1  omode=Inherit via internal rule  otype=sfix(16)  scale=2^-15  rndmethod=Unbiased  factor=1  satmethod=Symmetric  shift_vec=[0 1 2 -1]  value=2^(DSPB_MMSE_param.FS-1)+1  inPortNames=['+'; '+';]  outPortNames=[' ']  dspbaimage=dspba_prim.jpg  text=fprintf('%s', num2str(value));  style=Optimised  visibilities=8 + 1024  floatPrecision=float32_m23  version=20120820
  Const1 : DSPBAPrim/Const  primtype=const  nInputs=0  nOutputs=1  omode=boolean  otype=sfix(16)  scale=2^-15  rndmethod=Unbiased  factor=1  satmethod=Symmetric  shift_vec=[0 1 2 -1]  value=0  inPortNames=['+'; '+';]  outPortNames=[' ']  dspbaimage=dspba_prim.jpg  text=fprintf('%s', num2str(value));  style=Optimised  visibilities=8 + 1024  floatPrecision=float32_m23  version=20120820
  Counter : DSPBAPrim/Counter  primtype=counter  nInputs=1  nOutputs=1  omode=Inherit via internal rule  otype=ufix(16)  scale=2^-0  rndmethod=Unbiased  factor=1  satmethod=Symmetric  shift_vec=[0 1 2 -1]  value=[0 2^(DSPB_MMSE_param.FS-1)+2 1]  inPortNames=[' '; ' ';]  outPortNames=[' ']  dspbaimage=dspba_prim.jpg  text=fprintf('counter\n[%d %d %d]', value(1), value(2), value(3));  style=Optimised  visibilities=8 + 1024  version=20090407
  Mux : DSPBAPrim/Mux  primtype=mux  nInputs=evalAionMaskParam(gcb,'value',1)+1  nOutputs=1  omode=Inherit via internal rule  otype=sfix(16)  scale=2^-15  rndmethod=Unbiased  factor=1  satmethod=Symmetric  shift_vec=[0 1 2 -1]  value=2  inPortNames=['s '; 'd0'; 'd1'; 'd2'; 'd3'; 'd4'; 'd5'; 'd6'; 'd7'; 'd8'; 'd9';]  outPortNames=[' ']  dspbaimage=dspba_prim.jpg  text=fprintf('%s', primtype);  style=Optimised  visibilities=1032  version=20131025
  SampleDelay2 : DSPBAPrim/SampleDelay  primtype=sampdelay  nInputs=1  nOutputs=1  omode=Inherit via internal rule  otype=sfix(16)  scale=2^-15  rndmethod=Unbiased  factor=1  satmethod=Symmetric  shift_vec=[0 1 2 -1]  value=1  inPortNames=[' '; ' ';]  outPortNames=[' ']  dspbaimage=dspba_prim.jpg  text=dpoly(1, eye(1,value+1), 'z')  style=Optimised  visibilities=8 + 1024 + 2^17 + 2^18  flexible=off  slackgroup=0  augmented=0  version=20090407  advOptions=[]
  output : Outport
  wires:
  input/1 -> Mux/2
  Counter/1 -> CmpEQ/1
  Const/1 -> CmpEQ/2
  Mux/1 -> Counter/1
  CmpEQ/1 -> output/1, SampleDelay2/1
  SampleDelay2/1 -> Mux/1
  Const1/1 -> Mux/3

== system DSPB_MMSE/dut/MMSE_TOP/a_priori_snr/frame_fuse ==
  input : Inport
  CmpEQ : DSPBAPrim/CmpEQ  primtype=cmpeq  nInputs=2  nOutputs=1  omode=boolean  otype=sfix(16)  scale=2^-15  rndmethod=Unbiased  factor=1  satmethod=Symmetric  shift_vec=[0 1 2 -1]  value=0  inPortNames=[' '; ' ';]  outPortNames=[' ']  dspbaimage=dspba_prim.jpg  text=fprintf('==');  style=Optimised  visibilities=0  advOptions=[]  version=20130117
  Const : DSPBAPrim/Const  primtype=const  nInputs=0  nOutputs=1  omode=Inherit via internal rule  otype=sfix(16)  scale=2^-15  rndmethod=Unbiased  factor=1  satmethod=Symmetric  shift_vec=[0 1 2 -1]  value=2^(DSPB_MMSE_param.FS-1)+1  inPortNames=['+'; '+';]  outPortNames=[' ']  dspbaimage=dspba_prim.jpg  text=fprintf('%s', num2str(value));  style=Optimised  visibilities=8 + 1024  floatPrecision=float32_m23  version=20120820
  Const1 : DSPBAPrim/Const  primtype=const  nInputs=0  nOutputs=1  omode=boolean  otype=sfix(16)  scale=2^-15  rndmethod=Unbiased  factor=1  satmethod=Symmetric  shift_vec=[0 1 2 -1]  value=0  inPortNames=['+'; '+';]  outPortNames=[' ']  dspbaimage=dspba_prim.jpg  text=fprintf('%s', num2str(value));  style=Optimised  visibilities=8 + 1024  floatPrecision=float32_m23  version=20120820
  Counter : DSPBAPrim/Counter  primtype=counter  nInputs=1  nOutputs=1  omode=Inherit via internal rule  otype=ufix(16)  scale=2^-0  rndmethod=Unbiased  factor=1  satmethod=Symmetric  shift_vec=[0 1 2 -1]  value=[0 2^(DSPB_MMSE_param.FS-1)+2 1]  inPortNames=[' '; ' ';]  outPortNames=[' ']  dspbaimage=dspba_prim.jpg  text=fprintf('counter\n[%d %d %d]', value(1), value(2), value(3));  style=Optimised  visibilities=8 + 1024  version=20090407
  Mux : DSPBAPrim/Mux  primtype=mux  nInputs=evalAionMaskParam(gcb,'value',1)+1  nOutputs=1  omode=Inherit via internal rule  otype=sfix(16)  scale=2^-15  rndmethod=Unbiased  factor=1  satmethod=Symmetric  shift_vec=[0 1 2 -1]  value=2  inPortNames=['s '; 'd0'; 'd1'; 'd2'; 'd3'; 'd4'; 'd5'; 'd6'; 'd7'; 'd8'; 'd9';]  outPortNames=[' ']  dspbaimage=dspba_prim.jpg  text=fprintf('%s', primtype);  style=Optimised  visibilities=1032  version=20131025
  SampleDelay2 : DSPBAPrim/SampleDelay  primtype=sampdelay  nInputs=1  nOutputs=1  omode=Inherit via internal rule  otype=sfix(16)  scale=2^-15  rndmethod=Unbiased  factor=1  satmethod=Symmetric  shift_vec=[0 1 2 -1]  value=1  inPortNames=[' '; ' ';]  outPortNames=[' ']  dspbaimage=dspba_prim.jpg  text=dpoly(1, eye(1,value+1), 'z')  style=Optimised  visibilities=8 + 1024 + 2^17 + 2^18  flexible=off  slackgroup=0  augmented=0  version=20090407  advOptions=[]
  output : Outport
  wires:
  input/1 -> Mux/2
  Counter/1 -> CmpEQ/1
  Const/1 -> CmpEQ/2
  Mux/1 -> Counter/1
  CmpEQ/1 -> output/1, SampleDelay2/1
  SampleDelay2/1 -> Mux/1
  Const1/1 -> Mux/3

== system DSPB_MMSE/dut/MMSE_TOP/fft_output_adapter/counter2 ==
  en : Inport
  CmpEQ : DSPBAPrim/CmpEQ  primtype=cmpeq  nInputs=2  nOutputs=1  omode=boolean  otype=sfix(16)  scale=2^-15  rndmethod=Unbiased  factor=1  satmethod=Symmetric  shift_vec=[0 1 2 -1]  value=0  inPortNames=[' '; ' ';]  outPortNames=[' ']  dspbaimage=dspba_prim.jpg  text=fprintf('==');  style=Optimised  visibilities=0  advOptions=[]  version=20130117
  Const1 : DSPBAPrim/Const  primtype=const  nInputs=0  nOutputs=1  omode=Specify via dialog  otype=ufix(DSPB_MMSE_param.FS + 1)  scale=2^-0  rndmethod=Unbiased  factor=1  satmethod=Symmetric  shift_vec=[0 1 2 -1]  value=2^(DSPB_MMSE_param.FS)+1  inPortNames=['+'; '+';]  outPortNames=[' ']  dspbaimage=dspba_prim.jpg  text=fprintf('%s', num2str(value));  style=Optimised  visibilities=8 + 1024  floatPrecision=float32_m23  version=20120820
  Const2 : DSPBAPrim/Const  primtype=const  nInputs=0  nOutputs=1  omode=Specify via dialog  otype=ufix(DSPB_MMSE_param.FS + 1)  scale=2^-0  rndmethod=Unbiased  factor=1  satmethod=Symmetric  shift_vec=[0 1 2 -1]  value=2^(DSPB_MMSE_param.FS)  inPortNames=['+'; '+';]  outPortNames=[' ']  dspbaimage=dspba_prim.jpg  text=fprintf('%s', num2str(value));  style=Optimised  visibilities=8 + 1024  floatPrecision=float32_m23  version=20120820
  Const3 : DSPBAPrim/Const  primtype=const  nInputs=0  nOutputs=1  omode=boolean  otype=ufix(10)  scale=2^-0  rndmethod=Unbiased  factor=1  satmethod=Symmetric  shift_vec=[0 1 2 -1]  value=1  inPortNames=['+'; '+';]  outPortNames=[' ']  dspbaimage=dspba_prim.jpg  text=fprintf('%s', num2str(value));  style=Optimised  visibilities=8 + 1024  floatPrecision=float32_m23  version=20120820
  Const4 : DSPBAPrim/Const  primtype=const  nInputs=0  nOutputs=1  omode=Inherit via internal rule  otype=ufix(10)  scale=2^-0  rndmethod=Unbiased  factor=1  satmethod=Symmetric  shift_vec=[0 1 2 -1]  value=0  inPortNames=['+'; '+';]  outPortNames=[' ']  dspbaimage=dspba_prim.jpg  text=fprintf('%s', num2str(value));  style=Optimised  visibilities=8 + 1024  floatPrecision=float32_m23  version=20120820
  LoadableCounter : DSPBAPrim/LoadableCounter  primtype=loadablecounter  nInputs=5  nOutputs=1  omode=Specify via dialog  otype=ufix(DSPB_MMSE_param.FS+1)  scale=2^-0  rndmethod=Unbiased  factor=1  satmethod=Symmetric  shift_vec=[0 1 2 -1]  value=[0 2^(DSPB_MMSE_param.FS)+1 1]  inPortNames=['en';'ld';'i ';'s ';'m ']  outPortNames=[' ']  dspbaimage=dspba_prim.jpg  text=fprintf('loadable\ncounter\n[%d %d %d]', value(1), value(2), value(3));  style=Optimised  visibilities=8 + 1024  version=20090407
  SampleDelay : DSPBAPrim/SampleDelay  primtype=sampdelay  nInputs=1  nOutputs=1  omode=Inherit via internal rule  otype=sfix(16)  scale=2^-15  rndmethod=Unbiased  factor=1  satmethod=Symmetric  shift_vec=[0 1 2 -1]  value=1  inPortNames=[' '; ' ';]  outPortNames=[' ']  dspbaimage=dspba_prim.jpg  text=dpoly(1, eye(1,value+1), 'z')  style=Optimised  visibilities=8 + 1024 + 2^17 + 2^18  flexible=off  slackgroup=0  augmented=0  version=20090407  advOptions=[]
  count : Outport
  wires:
  Const2/1 -> CmpEQ/2
  CmpEQ/1 -> SampleDelay/1
  Const4/1 -> LoadableCounter/3
  Const1/1 -> LoadableCounter/5
  SampleDelay/1 -> LoadableCounter/2
  Const3/1 -> LoadableCounter/4
  en/1 -> LoadableCounter/1
  LoadableCounter/1 -> CmpEQ/1, count/1

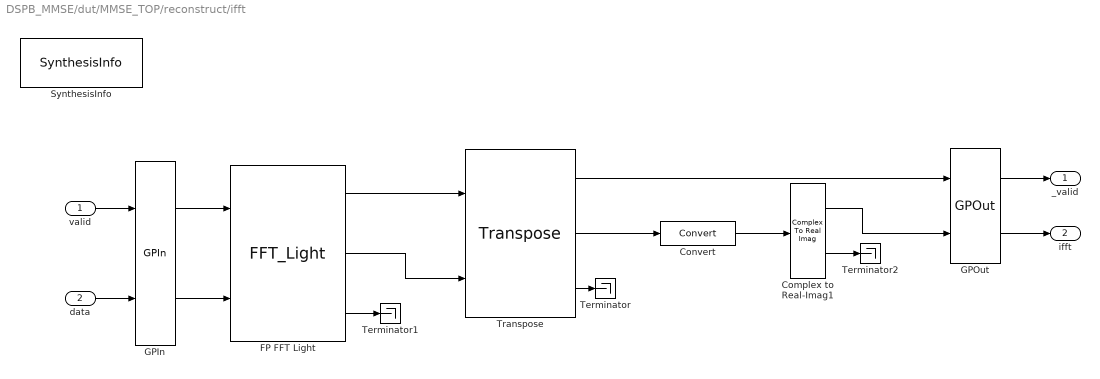
== system DSPB_MMSE/dut/MMSE_TOP/reconstruct/ifft ==
  valid : Inport
  data : Inport  Port=2
  Complex to Real-Imag1 : ComplexToRealImag
  Convert : DSPBAPrim/Convert  primtype=convert  nInputs=1  nOutputs=1  omode=single  otype=sfix(16)  scale=2^-15  rndmethod=Biased  factor=1  satmethod=None  shift_vec=[0 1 2 -1]  value=round([0:255]/17)  inPortNames=[' '; ' ';]  outPortNames=[' '; 'c']  dspbaimage=dspba_prim.jpg  text=fprintf('convert');  style=Optimised  visibilities=8+64+256+2^17  clipdetect=off  floatPrecision=float32_m23  advOptions=[]  version=20130211
  FP FFT Light : DspbAdvFftLibrary/Common/FFT_Light  IFFT=true  subchannels=1  br_in=false  N=DSPB_MMSE_param.FS  in_type=dspba.namedVPFloat('single')  type_strings=dspba.fft.all_float(DSPB_MMSE_param.FS,dspba.namedVPFloat('single'))  faithful=false  wirecount=1
  GPIn : DSPBAPrim/GPIn  primtype=gpin  nInputs=evalAionMaskParam(gcb,'value',1)  nOutputs=evalAionMaskParam(gcb,'value',1)  omode=Inherit via internal rule  otype=sfix(16)  scale=2^-15  rndmethod=Unbiased  factor=1  satmethod=Symmetric  shift_vec=[0 1 2 -1]  value=2  inPortNames=[' ' ' ' ' ' ' ' ' ' ' ' ' ' ' ' ' ' ' ' ' ' ' ' ' ' ' ' ' ' ' ' ' ' ' ' ' ' ' ' ' ' ' ' ' ' ' ' ' ' ' ' ' ' ' ' ' ' ' ' ' ' ' ' ' ' ' ' ' ']'  outPortNames=[' ' ' ' ' ' ' ' ' ' ' ' ' ' ' ' ' ' ' ' ' ' ' ' ' ' ' ' ' ' ' ' ' ' ' ' ' ' ' ' ' ' ' ' ' ' ' ' ' ' ' ' ' ' ' ' ' ' ' ' ' ' ' ' ' ' ' ' ' ']'  dspbaimage=dspba_prim.jpg  text=fprintf('GPIn');  style=Optimised  visibilities=1024  latencyCorrection=0  scheduleOrigin=on  version=20090407
  GPOut : DSPBAPrim/GPOut  primtype=gpout  nInputs=evalAionMaskParam(gcb,'value',1)  nOutputs=evalAionMaskParam(gcb,'value',1)  omode=Inherit via internal rule  otype=sfix(16)  scale=2^-15  rndmethod=Unbiased  factor=1  satmethod=Symmetric  shift_vec=[0 1 2 -1]  value=2  inPortNames=[' ' ' ' ' ' ' ' ' ' ' ' ' ' ' ' ' ' ' ' ' ' ' ' ' ' ' ' ' ' ' ' ' ' ' ' ' ' ' ' ' ' ' ' ' ' ' ' ' ' ' ' ' ' ' ' ' ' ' ' ' ' ' ' ' ' ' ' ' ']'  outPortNames=[' ' ' ' ' ' ' ' ' ' ' ' ' ' ' ' ' ' ' ' ' ' ' ' ' ' ' ' ' ' ' ' ' ' ' ' ' ' ' ' ' ' ' ' ' ' ' ' ' ' ' ' ' ' ' ' ' ' ' ' ' ' ' ' ' ' ' ' ' ']'  dspbaimage=dspba_prim.jpg  text=fprintf('GPOut');  style=Optimised  visibilities=1024  latencyCorrection=0  version=20090407
  SynthesisInfo : DSPBAPrim/SynthesisInfo  primtype=synthinfo  nInputs=0  nOutputs=0  omode=Inherit via internal rule  otype=sfix(16)  scale=2^-15  rndmethod=Truncate  factor=1  satmethod=Symmetric  shift_vec=[0 1 2 -1]  value=99  inPortNames=[' '; ' ';]  outPortNames=[' ']  dspbaimage=dspba_prim_ctrl.jpg  text=fprintf('Style=%s', style);  style=Scheduled  visibilities=32768  constraintInUse=off  constraintRelation=>  constraintLimit=2  bitAccurate=on  version=20150220
  Terminator : Terminator
  Terminator1 : Terminator
  Terminator2 : Terminator
  Transpose : DspbAdvFftLibrary/Common/Transpose  perm=[fliplr(0:DSPB_MMSE_param.FS-1)]
  _valid : Outport
  ifft : Outport  Port=2
  wires:
  Transpose/3 -> Terminator/1
  FP FFT Light/3 -> Terminator1/1
  valid/1 -> GPIn/1
  data/1 -> GPIn/2
  GPOut/1 -> _valid/1
  GPOut/2 -> ifft/1
  GPIn/1 -> FP FFT Light/1
  GPIn/2 -> FP FFT Light/2
  FP FFT Light/1 -> Transpose/1
  FP FFT Light/2 -> Transpose/2
  Transpose/2 -> Convert/1
  Convert/1 -> Complex to Real-Imag1/1
  Complex to Real-Imag1/2 -> Terminator2/1
  Complex to Real-Imag1/1 -> GPOut/2
  Transpose/1 -> GPOut/1
